simulink model "FINAL_AUTO_PHASE_1_V3"  (R2020b)
settings: Solver=ode23t  StartTime=0.0  StopTime=180.1  FixedStep=0.05  RelTol=1e-3  EnableMultiTasking=on
model workspace (MAT data in the model file):
  GRID_SIDE = 0.457142857143
  HALF_TICKS_TO_DIST = 0.00174532925
  LATCHER_OFFSET = 0.3934603175
  LATCH_CELL_TIME = 0.5
  LOWER_PLATFORM_TIME = 0.5
  SPACE_SIDE = 0.152380952381
  SURVEY_TURN_ANGLE = 22.7856177106
  WAIT_CONFIRM_CELL_TIME = 0.08
  mapForSim : object (value not decoded)
  occGrid : robotics.BinaryOccupancyGrid (value not decoded)
undefined symbols (not defined in the file): cellLevel, cellPose, cellTypeArray, FloorSurface, isoPoses, platformPoses, PlowSurface, Ref, RobotSurface, WallSurface, X, Y, Z
libraries: sm_lib x286, nesl_utility x157, simulink x72, pid_lib x3
(part 15 of 15)

== matlab function FINAL_AUTO_PHASE_1_V3/BEST Robotics 2020 Game (Double-Click)/Vaccines/Vaccine2/MATLAB Function1 ==
  settings: updateMethod=DISCRETE
  data: drop input; level input; objPoseX output; robotPoseX input; robotPoseY input; objPoseY output; vaccine output
function [objPoseX, objPoseY, vaccine] = latchObject(drop, level, robotPoseX, robotPoseY)
persistent stateX stateY stateZ prevDrop dropped
if isempty(stateX)
    stateX=robotPoseX+0.14;
    stateY=robotPoseY;
    stateZ=0.15;
    prevDrop=0;
    dropped=0;
end

if drop && prevDrop && ~dropped
    stateX=robotPoseX;
    stateY=robotPoseY;
    stateZ=level*0.4;
    objPoseX=robotPoseX;
    objPoseY=robotPoseY;
    dropped=1;
elseif dropped
    objPoseX=stateX;
    objPoseY=stateY;

else
    objPoseX=robotPoseX-0.11;
    objPoseY=robotPoseY+0.11;
end
prevDrop=drop;
vaccine=stateZ;

== stateflow chart FINAL_AUTO_PHASE_1_V3/stateflow MAIN_PROGRAM ==
  state MAIN_PROGRAM
    state sidesSurveyed = hasSurveyedSides(pivotSide) [function] [commented out]
    state PHASE_1
      state DROP_VAC_1
      state DROP_VAC_2
      state CLEAR_PLATFORM_1
      state DROP_VAC_3
      state CLEAR_PLATFORM_2
      (default) -> DROP_VAC_1
      DROP_VAC_1 -> DROP_VAC_2 : [hasDroppedVacAt(0.9904761905, 0.8380952381)]
      DROP_VAC_2 -> CLEAR_PLATFORM_1 : [hasDroppedVacAt(1.0404761905, 2.361904762)]
      CLEAR_PLATFORM_1 -> DROP_VAC_3 : [hasClearedPlatformAt(5, 5)]
      DROP_VAC_3 -> CLEAR_PLATFORM_2 : [hasDroppedVacAt(2.361904762, 1.752380952)]
    state PAHSE_2
      state EVACUATE_UNINFECTED_CELLS
      state FINISHED_AUTONOMOUS
        entry:
        leftMotor = 0
        rightMotor = 0
      (default) -> EVACUATE_UNINFECTED_CELLS
      EVACUATE_UNINFECTED_CELLS -> FINISHED_AUTONOMOUS : [hasSavedAllUninfected()]
    state ? [function] [commented out]
    state deliveredVac = hasDroppedVacAt(xCoord, yCoord) [function]
    state platformCleared = hasClearedPlatformAt(gridX,gridY) [function]
    state allUninfectedSaved = hasSavedAllUninfected [function]
    (default) -> PHASE_1
    CLEAR_PLATFORM_2 -> PAHSE_2 : [hasClearedPlatformAt(6, 0)]
  (default) -> MAIN_PROGRAM
  data: pivotSide function_input double size=1; sidesSurveyed function_output double size=1; xCoord function_input double size=1; yCoord function_input double size=1; deliveredVac function_output; gridX function_input double size=1; gridY function_input double size=1; platformCleared function_output; allUninfectedSaved function_output; rightMotor data_store_memory; leftMotor data_store_memory

== matlab function FINAL_AUTO_PHASE_1_V3/BEST Robotics 2020 Game (Double-Click)/Vaccines/Vaccine1/MATLAB Function1 ==
  settings: updateMethod=DISCRETE
  data: drop input; level input; objPoseX output; robotPoseX input; robotPoseY input; objPoseY output; vaccine output
function [objPoseX, objPoseY, vaccine] = latchObject(drop, level, robotPoseX, robotPoseY)
persistent stateX stateY stateZ prevDrop dropped
if isempty(stateX)
    stateX=robotPoseX+0.14;
    stateY=robotPoseY;
    stateZ=0.15;
    prevDrop=0;
    dropped=0;
end

if drop && prevDrop && ~dropped
    stateX=robotPoseX;
    stateY=robotPoseY;
    stateZ=level*0.4;
    objPoseX=robotPoseX;
    objPoseY=robotPoseY;
    dropped=1;
elseif dropped
    objPoseX=stateX;
    objPoseY=stateY;

else
    objPoseX=robotPoseX-0.11;
    objPoseY=robotPoseY-0.11;
end
prevDrop=drop;
vaccine=stateZ;

== matlab function FINAL_AUTO_PHASE_1_V3/function getFullRobotAngle ==
  data: robotAngle input; fullRobotAngle input; fullRobotAngle output; leftTicks input; rightTicks input; prevLTicks input; prevRTicks input
function fullRobotAngle = getFullRobotAngle(robotAngle, fullRobotAngle, ...
    leftTicks, rightTicks, prevLTicks, prevRTicks)

% just choose one of the encoder tick differences, since
    % the motors always have the same speed
% the weird decimal is the change in degrees per encoder tick
angleChange = abs(leftTicks - prevLTicks) * 0.7804878049;

% if the robot is turning clockwise
if leftTicks > prevLTicks && rightTicks < prevRTicks
    fullRobotAngle = fullRobotAngle - angleChange;
% if the robot is turning counter-clockwise
elseif rightTicks > prevRTicks && leftTicks < prevLTicks
    fullRobotAngle = fullRobotAngle + angleChange;
end

% normalize the angle to be 0 to 359 degrees
if fullRobotAngle >= 360
    fullRobotAngle = mod(fullRobotAngle, 360);
elseif fullRobotAngle < 0
    fullRobotAngle = fullRobotAngle + 360;
end

% last-minute (ngl kinda janky) angle correction 
if abs(fullRobotAngle - robotAngle) ... 
        < abs(fullRobotAngle - (360 - robotAngle))
    fullRobotAngle = robotAngle;
else
    fullRobotAngle = 360 - robotAngle;
end

== stateflow chart FINAL_AUTO_PHASE_1_V3/stateflow MAIN_PROGRAM/MAIN_PROGRAM.hasDroppedVacAt/Stateflow ==
  state DROP_VACCINE
    entry:
    leftMotor = 0
    rightMotor = 0
    dropVaccine()
    vaccineDropped = true
  state MOVE_TO_VAC_SQUARE
    entry:
    vaccineDropped = false
  (default) -> MOVE_TO_VAC_SQUARE
  MOVE_TO_VAC_SQUARE -> DROP_VACCINE : [hasMovedToCoords(xCoord, yCoord, 0)]
  DROP_VACCINE -> MOVE_TO_VAC_SQUARE
  data: xCoord input; yCoord input; vaccineDropped output; leftMotor data_store_memory; rightMotor data_store_memory

== matlab function FINAL_AUTO_PHASE_1_V3/stateflow MAIN_PROGRAM/MAIN_PROGRAM.hasClearedPlatformAt/function getCellSurveyPivots/function getCellSurveyCheckpoints ==
  data: gridX input; pivotSide output; gridY input double; startPivotPoint output; finalPoint output; GRID_SIDE parameter double size=1; SPACE_SIDE parameter size=1; xPos data_store_memory; yPos data_store_memory; LATCHER_OFFSET parameter
function [pivotSide,startPivotPoint,finalPoint] ...
    = getCellSurveyPivots(gridX,gridY, GRID_SIDE, SPACE_SIDE, LATCHER_OFFSET)

global xPos;
global yPos;

% note that the entire coordinate system represented in this code has
% been rotated by -45 degrees (45 degrees clockwise) to logically
% decide if the robot is closer to the top, bottom, left, or right
% edge of the target grid-square

% with our rotated coord. system, make the center of the grid-square the
% relative origin for easy quadrant case logic

% centerX and centerY are the grid-square's center non-rotated coords.
centerX = (gridX + 0.5) * GRID_SIDE;
centerY = (gridY + 0.5) * GRID_SIDE;

[originX, originY] = clockwise45Rotate( ...
    centerX, ...
    centerY);

[rotXPos, rotYPos] = clockwise45Rotate( ...
    xPos, yPos);

orthPivotDist = sqrt(LATCHER_OFFSET^2 - SPACE_SIDE^2);

% is in quadrant one
if rotXPos > originX && rotYPos >= originY
    pivotSide = 1;
    startPivotPoint = [ ...
        centerX + SPACE_SIDE + orthPivotDist ...
        centerY];
    finalPoint = [ ...
        centerX - SPACE_SIDE + LATCHER_OFFSET ...
        centerY];
    
% is in quadrant two
elseif rotXPos <= originX && rotYPos > originY
    pivotSide = 2;
    startPivotPoint = [ ...
        centerX ...
        centerY + SPACE_SIDE + orthPivotDist];
    finalPoint = [ ...
        centerX ...
        centerY - SPACE_SIDE + LATCHER_OFFSET];
    
% is in quadrant three
elseif rotXPos < originX && rotYPos <= originY
    pivotSide = 3;
    startPivotPoint = [ ...
        centerX - SPACE_SIDE - orthPivotDist ...
        centerY];
    finalPoint = [ ...
        centerX + SPACE_SIDE - LATCHER_OFFSET ...
        centerY];
    
% is in quadrant four
else % xPos >= centerX && yPos < centerY
    pivotSide = 4;
    startPivotPoint = [ ...
        centerX ...
        centerY - SPACE_SIDE - orthPivotDist];
    finalPoint = [ ...
        centerX ...
        centerY + SPACE_SIDE - LATCHER_OFFSET];
    
end

== stateflow chart FINAL_AUTO_PHASE_1_V3/function hasTurnedToAngle/stateflow integrateSettleTime ==
  state ELAPSE_SETTLE_TIME
    during:
    settledTime = settledTime + 1
  state RESET_SETTLE_TIME
    entry:
    settledTime = 0
  (default) -> RESET_SETTLE_TIME
  RESET_SETTLE_TIME -> ELAPSE_SETTLE_TIME : [error <= TOLERANCE]
  ELAPSE_SETTLE_TIME -> RESET_SETTLE_TIME : [error > TOLERANCE]
  data: TOLERANCE input; error input; settledTime data_store_memory

== stateflow chart FINAL_AUTO_PHASE_1_V3/function hasMovedToCoords/stateflow hasMovedToCoords ==
  state CALCULATE_PATH
    entry:
    hasArrived = false
    changeX = xCoord - xPos
    changeY = yCoord - yPos
    targetAngle = normalizeAngle(...
    atand(changeY / changeX), changeX)
    wantedDist = getDist(changeX, changeY, useRobotPos)
    oldXCoord = xCoord
    oldYCoord = yCoord
  state TURN_TO_TARGET
  state DRIVE_TO_TARGET
  state HAS_ARRIVED
    entry: hasArrived = true
  (default) -> CALCULATE_PATH
  CALCULATE_PATH -> TURN_TO_TARGET
  TURN_TO_TARGET -> DRIVE_TO_TARGET : [hasTurnedToAngle(targetAngle)]
  DRIVE_TO_TARGET -> HAS_ARRIVED : [hasMovedDist(wantedDist)]
  HAS_ARRIVED -> CALCULATE_PATH : [xCoord ~= oldXCoord || yCoord ~= oldYCoord]
  data: angle function_output; angle function_input; xChange function_input; targetDist function_output double size=1; xChange function_input; yChange function_input; usingRobotPos function_input; LATCHER_OFFSET parameter size=1; xCoord input; yCoord input; targetAngle local; xPos data_store_memory; yPos data_store_memory; hasArrived output; oldYCoord local; oldXCoord local; changeY local; changeX local; useRobotPos input; wantedDist local
  function angle = normalizeAngle(angle, xChange):
    | function angle = normalizeAngle(angle, xChange)
    | 
    | if xChange < 0
    |     angle = angle + 180;
    | end
  function targetDist = getDist(xChange, yChange, usingRobotPos):
    | function targetDist = getDist(xChange, yChange, usingRobotPos)
    |  
    | targetDist = sqrt(xChange^2 + yChange^2);
    | 
    | if ~usingRobotPos
    |     % the weird decimal is the constant distance 
    |     % between the latcher xy and the robot xy
    |     targetDist = targetDist - LATCHER_OFFSET;
    | end

== stateflow chart FINAL_AUTO_PHASE_1_V3/function hasMovedDist/stateflow postSettleDist ==
  state SETTLE
  state RESET_DIST_AFTER_SETTLE
    entry:
    leftMotor = 0
    rightMotor = 0
    resetLeftEncoder = 1
    resetRightEncoder = 1
    straightDistTraveled = 0
    resetLeftEncoder = 0
    resetRightEncoder = 0
  (default) -> SETTLE
  RESET_DIST_AFTER_SETTLE -> SETTLE
  SETTLE -> RESET_DIST_AFTER_SETTLE : [distHasSettled]
  data: distHasSettled input; resetLeftEncoder data_store_memory; resetRightEncoder data_store_memory; straightDistTraveled data_store_memory; leftMotor data_store_memory; rightMotor data_store_memory

== matlab function FINAL_AUTO_PHASE_1_V3/function hasMovedDist/function getMoveDirSign ==
  data: u input double size=1; sign output double size=1
function sign = getMoveDirSign(u)

if u > 0
    sign = 1;
elseif u < 0
    sign = -1;
else
    sign = 0;
end

== stateflow chart FINAL_AUTO_PHASE_1_V3/function hasMovedDist/stateflow integrateSettleTime ==
  state ELAPSE_SETTLE_TIME
    during:
    settledTime = settledTime + 1
  state RESET_SETTLE_TIME
    entry:
    settledTime = 0
  (default) -> RESET_SETTLE_TIME
  RESET_SETTLE_TIME -> ELAPSE_SETTLE_TIME : [error <= TOLERANCE]
  ELAPSE_SETTLE_TIME -> RESET_SETTLE_TIME : [error > TOLERANCE]
  data: TOLERANCE input; error input; settledTime data_store_memory

== stateflow chart FINAL_AUTO_PHASE_1_V3/stateflow MAIN_PROGRAM/MAIN_PROGRAM.hasDroppedVacAt/function dropVaccine/stateflow dropVaccine ==
  (default) -> (junction 11)
  (junction 11) -> (junction 12) [order 1] : [all((vaccineReleases == [0 0 0]) == 1)]
  (junction 11) -> (junction 13) [order 2]
  (junction 12) -> (junction 17) : {vaccineReleases = [1 0 0];}
  (junction 13) -> (junction 14) [order 1] : [all((vaccineReleases == [1 0 0]) == 1)]
  (junction 13) -> (junction 15) [order 2] : {vaccineReleases = [1 1 1];}
  (junction 14) -> (junction 16) : {vaccineReleases = [1 1 0];}
  (junction 16) -> (junction 15)
  (junction 17) -> (junction 16)
  data: vaccineReleases data_store_memory

== matlab function FINAL_AUTO_PHASE_1_V3/stateflow MAIN_PROGRAM/MAIN_PROGRAM.hasClearedPlatformAt/function clockwise45Rotate/function clockwise45Rotate ==
  data: oldX input; rotatedX output; oldY input; rotatedY output
function [rotatedX,rotatedY] = clockwise45Rotate(oldX,oldY)

rotatedX = oldX*cosd(45) - oldY*sind(45);
rotatedY = oldX*sin(45) + oldY*cosd(45);

== matlab function FINAL_AUTO_PHASE_1_V3/function getCoordChanges ==
  data: changeInDist input; fullRobotAngle input; newXPos output; newYPos output; xPos data_store_memory; yPos data_store_memory
function [newXPos, newYPos] = updateCoords(changeInDist, fullRobotAngle)
% assumes that the robot angle input is from 0 to 360 degrees

global xPos;
global yPos;

newXPos = xPos + (changeInDist * cosd(fullRobotAngle));
newYPos = yPos + (changeInDist * sind(fullRobotAngle));

== stateflow chart FINAL_AUTO_PHASE_1_V3/stateflow MAIN_PROGRAM/MAIN_PROGRAM.hasClearedPlatformAt/Stateflow1 ==
  state INIT_AND_CALC_CHECKPOINTS
    entry:
    platformCleared = false
    [startPoint, firstDiagEnd, lateralEnd, secondDiagEnd, stopPoint] ...
    = getCellSurveyCheckpoints(gridX, gridY)
  state RAISE_LATCHER
    entry:
    scoringLevel = 1
  state START_POINT
  state FIRST_DIAG_POINT
  state DROP_CELL
    entry:
    scoringLevel = 0
    latchCell = 0
    platformCleared = true
  state PLATFORM_CELL_FOUND
    entry:
    leftMotor = 0
    rightMotor = 0
    latchCell = 1
  state CONFIRM_CELL
  state LATERAL_POINT
  state SECOND_DIAG_POINT
  state STOP_POINT
  (default) -> INIT_AND_CALC_CHECKPOINTS
  DROP_CELL -> INIT_AND_CALC_CHECKPOINTS
  STOP_POINT -> INIT_AND_CALC_CHECKPOINTS [order 2]
  INIT_AND_CALC_CHECKPOINTS -> RAISE_LATCHER : [after(0.25, sec)]
  RAISE_LATCHER -> START_POINT : [hasMovedToCoords(startPoint(1), startPoint(2), 1)]
  START_POINT -> CONFIRM_CELL [order 2] : [~isnan(detectedCellType)]
  START_POINT -> FIRST_DIAG_POINT [order 1] : [hasMovedToCoords(firstDiagEnd(1), firstDiagEnd(2), 1)]
  FIRST_DIAG_POINT -> CONFIRM_CELL [order 2] : [~isnan(detectedCellType)]
  FIRST_DIAG_POINT -> LATERAL_POINT [order 1] : [hasMovedToCoords(lateralEnd(1), lateralEnd(2), 1)]
  SECOND_DIAG_POINT -> CONFIRM_CELL [order 2] : [~isnan(detectedCellType)]
  CONFIRM_CELL -> PLATFORM_CELL_FOUND : [after(0.05, sec)]
  STOP_POINT -> CONFIRM_CELL [order 1] : [~isnan(detectedCellType)]
  LATERAL_POINT -> CONFIRM_CELL [order 2] : [~isnan(detectedCellType)]
  PLATFORM_CELL_FOUND -> DROP_CELL : [after(0.75, sec)]
  LATERAL_POINT -> SECOND_DIAG_POINT [order 1] : [hasMovedToCoords(secondDiagEnd(1), secondDiagEnd(2), 1)]
  SECOND_DIAG_POINT -> STOP_POINT [order 1] : [hasMovedToCoords(stopPoint(1), stopPoint(2), 1)]
  data: stopPoint local; startPoint local; secondDiagEnd local; lateralEnd local; firstDiagEnd local; gridX input; gridY input; scoringLevel data_store_memory; platformCleared output; detectedCellType data_store_memory; latchCell data_store_memory; leftMotor data_store_memory; rightMotor data_store_memory
